simulink model "Stinger"  (R2023a)
settings: Solver=VariableStepAuto  StartTime=0.0  StopTime=20  FixedStep=1e-3  EnableMultiTasking=on
values from neighbouring files (symbols this model uses):
  bp = 0.001    [ControlLawsScript.m]    (also in ControlLaws_Script.m)
  bq = 0.001    [ControlLawsScript.m]    (also in ControlLaws_Script.m)
  br = 0.001    [ControlLawsScript.m]    (also in ControlLaws_Script.m)
  cx = 5    [ControlLawsScript.m]    (also in ControlLaws_Script.m)
  cy = 5    [ControlLawsScript.m]    (also in ControlLaws_Script.m)
  cz = 5    [ControlLawsScript.m]    (also in ControlLaws_Script.m)
  g = 9.80665    [ControlLawsScript.m]    (also in ControlLaws_Script.m; Qball_X8_Model.m = 9.87)
  Kp = (Jx/Tc)-bp    (= 1.02772632451)    [ControlLawsScript.m]    (also in ControlLaws_Script.m = 4.11390529802)
  Kp2 = Jx*((4/ts))*((-4/ts)+((bp+Kp)/Jx))/Kp    (= 1.68163467643)    [ControlLawsScript.m]    (also in ControlLaws_Script.m = 6.72163348437)
  Kq = (Jy/Tc)-bq    (= 1.02971502036)    [ControlLawsScript.m]    (also in ControlLaws_Script.m = 4.12186008142)
  Kq2 = Jy*((4/ts))*((-4/ts)+((bq+Kq)/Jy))/Kq    (= 1.68163151937)    [ControlLawsScript.m]    (also in ControlLaws_Script.m = 6.72163033191)
  Kr = (Jz/Tc)-br    (= 1.98490876719)    [ControlLawsScript.m]    (also in ControlLaws_Script.m = 7.94263506876)
  Kr2 = Jz*((4/ts))*((-4/ts)+((br+Kr)/Jz))/Kr    (= 1.68084638651)    [ControlLawsScript.m]    (also in ControlLaws_Script.m = 6.72084606682)
  kv = 1/930    (= 0.0010752688172)    [StingerScript.m]
  Kx = abs(Kx)    [ControlLawsScript.m]    (also in ControlLaws_Script.m)
  Ky = abs(Ky)    [ControlLawsScript.m]    (also in ControlLaws_Script.m)
  Kz = (m/Tcz)-cz    (= 38.5143536865)    [ControlLawsScript.m]    (also in ControlLaws_Script.m)
  Kz2 = m*((4/tsz))*((-4/tsz)+((cz+Kz)/m))/Kz    (= 1.89810050529)    [ControlLawsScript.m]    (also in ControlLaws_Script.m)
  m = 3.4811482949175    (= 3.48114829492)    [ControlLawsScript.m]    (also in ControlLaws_Script.m; Qball_X8_Model.m = 1.45)
  pitch_angle_limit = pi/6    (= 0.523598775598)    [ControlLawsScript.m]    (also in ControlLaws_Script.m = 0.558505360638)
  R2D = 180/pi    (= 57.2957795131)    [ControlLawsScript.m]    (also in ControlLaws_Script.m)
  roll_angle_limit = pi/6    (= 0.523598775598)    [ControlLawsScript.m]    (also in ControlLaws_Script.m = 0.558505360638)
  z_x = cx    (= 5)    [ControlLawsScript.m]    (also in ControlLaws_Script.m)
  z_y = cy    (= 5)    [ControlLawsScript.m]    (also in ControlLaws_Script.m)
undefined symbols (not defined in the file or in its folder): FC, LAC, LeftAftArm, LeftAftProp, LeftAftSkid, LeftArm, LeftFrontArm, LeftFrontProp, LeftFrontSkid, LeftProp, Lower, missionPlanX, missionPlanY, missionPlanYaw, missionPlanZ, RAC, RightAftArm, RightAftProp, RightAftSkid, RightArm, RightFrontArm, RightFrontProp, RightFrontSkid, RightProp, SC, timeConstant, Upper, X, Y, Z
libraries: sm_lib x98, nesl_utility x56, fl_lib x45, ee_lib x19, batteryecm_lib x2, sharedtransformsys x1, sharedutil x1
(part 4 of 4)

== matlab function Stinger/PLANT MODEL/ELECTRIC SYSTEM/Motor 1/RPM to Resistive Torque and Thrust1/Thrust & Torque Based on Propeller Rotational and Translational Velocity ==
  data: Thrust output; Velocity input; RPM input; Torque output
function [Thrust,Torque]= fcn(Velocity, RPM)

%Thrust

s1 = 0.007241;
s2 = -7.12e-05;
s3 = -0.00219;
s4 = -1.683e-05;
s5 = 1.619e-07;
Thrust = s1*Velocity + s2*RPM + s3*Velocity.^2 + s4*Velocity.*RPM + s5*RPM.^2;

%Torque

k1 = 0.000295;
k2 = -1.33e-07;
k3 = -7.089e-05;
k4 = 7.352e-08;
k5 = 2.21e-09;
Torque = k1*Velocity + k2*RPM + k3*Velocity.^2 + k4*Velocity.*RPM + k5*RPM.^2;

== matlab function Stinger/PLANT MODEL/ELECTRIC SYSTEM/Motor 4/RPM to Resistive Torque and Thrust/Thrust & Torque Based on Propeller Rotational and Translational Velocity ==
  data: Thrust output; Velocity input; RPM input; Torque output
function [Thrust,Torque]= fcn(Velocity, RPM)

%Thrust

s1 = 0.007241;
s2 = -7.12e-05;
s3 = -0.00219;
s4 = -1.683e-05;
s5 = 1.619e-07;
Thrust = s1*Velocity + s2*RPM + s3*Velocity.^2 + s4*Velocity.*RPM + s5*RPM.^2;

%Torque

k1 = 0.000295;
k2 = -1.33e-07;
k3 = -7.089e-05;
k4 = 7.352e-08;
k5 = 2.21e-09;
Torque = k1*Velocity + k2*RPM + k3*Velocity.^2 + k4*Velocity.*RPM + k5*RPM.^2;

== matlab function Stinger/PLANT MODEL/ELECTRIC SYSTEM/Motor 5/RPM to Resistive Torque and Thrust/Thrust & Torque Based on Propeller Rotational and Translational Velocity ==
  data: Thrust output; Velocity input; RPM input; Torque output
function [Thrust,Torque]= fcn(Velocity, RPM)

%Thrust

s1 = 0.007241;
s2 = -7.12e-05;
s3 = -0.00219;
s4 = -1.683e-05;
s5 = 1.619e-07;
Thrust = s1*Velocity + s2*RPM + s3*Velocity.^2 + s4*Velocity.*RPM + s5*RPM.^2;

%Torque

k1 = 0.000295;
k2 = -1.33e-07;
k3 = -7.089e-05;
k4 = 7.352e-08;
k5 = 2.21e-09;
Torque = k1*Velocity + k2*RPM + k3*Velocity.^2 + k4*Velocity.*RPM + k5*RPM.^2;

== matlab function Stinger/PLANT MODEL/ELECTRIC SYSTEM/Motor 2/RPM to Resistive Torque and Thrust/Thrust & Torque Based on Propeller Rotational and Translational Velocity ==
  data: Thrust output; Velocity input; RPM input; Torque output
function [Thrust,Torque]= fcn(Velocity, RPM)

%Thrust

s1 = 0.007241;
s2 = -7.12e-05;
s3 = -0.00219;
s4 = -1.683e-05;
s5 = 1.619e-07;
Thrust = s1*Velocity + s2*RPM + s3*Velocity.^2 + s4*Velocity.*RPM + s5*RPM.^2;

%Torque

k1 = 0.000295;
k2 = -1.33e-07;
k3 = -7.089e-05;
k4 = 7.352e-08;
k5 = 2.21e-09;
Torque = k1*Velocity + k2*RPM + k3*Velocity.^2 + k4*Velocity.*RPM + k5*RPM.^2;

== matlab function Stinger/PLANT MODEL/ELECTRIC SYSTEM/Motor 6/RPM to Resistive Torque and Thrust/Thrust & Torque Based on Propeller Rotational and Translational Velocity ==
  data: Thrust output; Velocity input; RPM input; Torque output
function [Thrust,Torque]= fcn(Velocity, RPM)

%Thrust

s1 = 0.007241;
s2 = -7.12e-05;
s3 = -0.00219;
s4 = -1.683e-05;
s5 = 1.619e-07;
Thrust = s1*Velocity + s2*RPM + s3*Velocity.^2 + s4*Velocity.*RPM + s5*RPM.^2;

%Torque

k1 = 0.000295;
k2 = -1.33e-07;
k3 = -7.089e-05;
k4 = 7.352e-08;
k5 = 2.21e-09;
Torque = k1*Velocity + k2*RPM + k3*Velocity.^2 + k4*Velocity.*RPM + k5*RPM.^2;

== matlab function Stinger/PLANT MODEL/ELECTRIC SYSTEM/Motor 3/RPM to Resistive Torque and Thrust/Thrust & Torque Based on Propeller Rotational and Translational Velocity ==
  data: Thrust output; Velocity input; RPM input; Torque output
function [Thrust,Torque]= fcn(Velocity, RPM)

%Thrust

s1 = 0.007241;
s2 = -7.12e-05;
s3 = -0.00219;
s4 = -1.683e-05;
s5 = 1.619e-07;
Thrust = s1*Velocity + s2*RPM + s3*Velocity.^2 + s4*Velocity.*RPM + s5*RPM.^2;

%Torque

k1 = 0.000295;
k2 = -1.33e-07;
k3 = -7.089e-05;
k4 = 7.352e-08;
k5 = 2.21e-09;
Torque = k1*Velocity + k2*RPM + k3*Velocity.^2 + k4*Velocity.*RPM + k5*RPM.^2;

== matlab function Stinger/CONTROL ALLOCATION/Control Allocation ==
  data: T input; w1 output; Mp input; Mq input; Mr input; w2 output; w3 output; w4 output; w5 output; w6 output
%% Control Allocation
function [w1,w2,w3,w4,w5,w6] = fcn(T,Mp,Mq,Mr)
rho = 1.293;         %Air density (kg/m^3)
d = 0.254;           %Diameter of propeller (m)
Ct = 0.0025*rho*d^4; %Thrust Coefficient
Cr=1.5925e-06;

% Cr = 0.001058;       %Torque coefficient (N/rad/s)
l=0.4;               %Arm length (m)

B=[ Ct,              Ct,         Ct,              Ct,                Ct,          Ct;
    Ct*l/2,          Ct*l,       Ct*l/2,         -Ct*l/2,           -Ct*l,       -Ct*l/2;
   -Ct*l*sqrt(3)/2,  0,          Ct*l*sqrt(3)/2,  Ct*l*sqrt(3)/2,    0,          -Ct*l*sqrt(3)/2;
    Cr,             -Cr,         Cr,             -Cr,                Cr,         -Cr];
Bi=pinv(B);
A=[T;Mq;Mp;Mr];
C=Bi*A;

c1=C(1); %Angular speed motor 1 (rpm)
c2=C(2);
c3=C(3);
c4=C(4);
c5=C(5);
c6=C(6);

c1 = max(c1, 0);
c2 = max(c2, 0);
c3 = max(c3, 0);
c4 = max(c4, 0);
c5 = max(c5, 0);
c6 = max(c6, 0);
    
w1 = sqrt(c1)*9.549;
w2 = sqrt(c2)*9.549;
w3 = sqrt(c3)*9.549;
w4 = sqrt(c4)*9.549;
w5 = sqrt(c5)*9.549;
w6 = sqrt(c6)*9.549;

== matlab function Stinger/Trajectory/Trajectory Control ==
  settings: updateMethod=DISCRETE
  data: xPosition output; missionPlanX input; missionPlanY input; missionPlanZ input; missionPlanYaw input; timeConstant input; yPosition output; zPosition output; simulationTime input; yaw output
function [xPosition, yPosition, zPosition, yaw] = fcn(missionPlanX, missionPlanY, missionPlanZ, missionPlanYaw, timeConstant, simulationTime)
    persistent prevX prevY prevZ prevYaw index startTime
    if isempty(prevX)
        % Initialize the previous position, yaw, index, and timer variables
        prevX = missionPlanX(1);
        prevY = missionPlanY(1);
        prevZ = missionPlanZ(1);
        prevYaw = missionPlanYaw(1);
        index = 1;
        startTime = simulationTime;  % Record the start time
    end
    
    % Get the number of points in the mission plan
    numPoints = numel(missionPlanX);
    
    % Wrap the index within the valid range of the mission plan matrices
    if index > numPoints
        % Output the last position and yaw as signals
        xPosition = prevX;
        yPosition = prevY;
        zPosition = prevZ;
        yaw = prevYaw;
        return; % Exit the function
    end
    
    % Get the current position and yaw from the mission plan matrices
    currX = missionPlanX(index);
    currY = missionPlanY(index);
    currZ = missionPlanZ(index);
    currYaw = missionPlanYaw(index);
    
    % Calculate the Euclidean distance
    distance = sqrt((currX - prevX)^2 + (currY - prevY)^2 + (currZ - prevZ)^2);
    
    % Calculate the delay time
    delay = distance * timeConstant;
    
    % Check if the elapsed time is less than the scaled delay
    elapsedTime = simulationTime - startTime;
    
    if elapsedTime < delay
        % Output the previous position and yaw as long as the delay is not reached
        xPosition = prevX;
        yPosition = prevY;
        zPosition = prevZ;
        yaw = prevYaw;
    else
        % Update the previous position and yaw
        prevX = currX;
        prevY = currY;
        prevZ = currZ;
        prevYaw = currYaw;
        
        % Update the index for the next point
        index = index + 1;
        
        % Reset the start time for the next delay
        startTime = simulationTime;
        
        % Output the current position and yaw
        xPosition = currX;
        yPosition = currY;
        zPosition = currZ;
        yaw = currYaw;
    end
end
